simulink model "Sepic"  (R2019b)
settings: Solver=VariableStepAuto  StartTime=0.0  StopTime=0.02  RelTol=1e-7  AbsTol=1e-7
values from neighbouring files (symbols this model uses):
  HPFenable = 1    [SimMain.m]
  Ilim_sepic = 3.5    [SimMain.m]
  Ki_sepic = 1.1    [SimMain.m]
  Ku_sepic = 1    [SimMain.m]
  R1_sepic = 1    [SimMain.m]
  RL_sepic = 200    [SimMain.m]
  tau_PI_sepic = 0.5e-3    (= 0.0005)    [SimMain.m]
  U2_sepic = 20    [SimMain.m]
  w_Amplitude = 0.3    [SimMain.m]
libraries: fl_lib x14, nesl_utility x12, ee_lib x11, simulink x2, powerlib_meascontrol x2
settings Model: Creator=Job  LastModifiedBy=Job
settings SolverCC: AlgebraicLoopSolver=LineSearch  PositivePriorityOrder=on

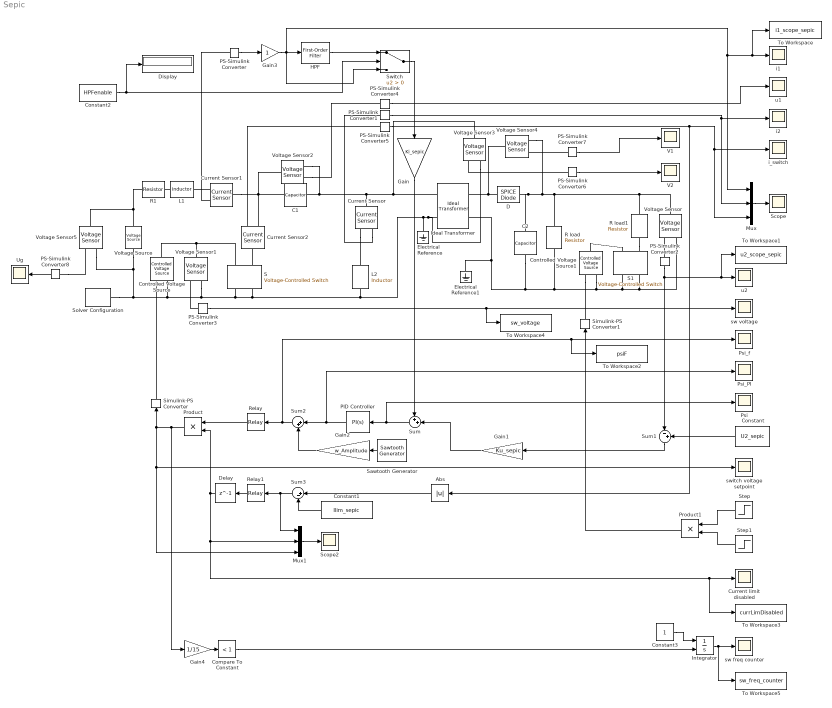
== system Sepic ==
  Abs : Abs
  C1 : ee_lib/Passive/Capacitor  cap_option=0  c=C1_sepic F  Cvec=[1e-05, 1e-06] F  Vvec=[0, 10] V  CV_table_symmetry=1  f_vec=[1, 10] kHz  DFext_vec=[.8, 1.2]  C_tol=0  enable_C_tol=0  tol_distribution=1  nSigma=4  r=1e-6 Ohm  g=0 1/Ohm  averaging_period=0 s  enable_operating_limits=0  operating_limit_action=2  max_working_voltage_range=[-25, 25] V  power_rating=1 W  enable_faults=0  fault_action=1  Cscale_faulted=100  R_faulted=1e-3 Ohm  G_faulted=0 1/Ohm  tau_fault=1e-3 s  enable_temporal_fault=0  t_fault=1 s  enable_behavioral_fault=0  max_permissible_voltage_range=[-100, 100] V  t_fail_on_voltage=1 s  i_specify=off  i_priority=None  i=0 A  i_nominal_specify=off  i_nominal_unit=A  i_nominal_value=1  v_specify=off  v_priority=None  v=0 V  v_nominal_specify=off  v_nominal_unit=V  v_nominal_value=1  vc_specify=off  vc_priority=High  vc=0 V  vc_nominal_specify=off  vc_nominal_unit=V  vc_nominal_value=1
      settings: SourceProductName=Simscape Electrical
  C2 : ee_lib/Passive/Capacitor  cap_option=0  c=C2_sepic F  Cvec=[1e-05, 1e-06] F  Vvec=[0, 10] V  CV_table_symmetry=1  f_vec=[1, 10] kHz  DFext_vec=[.8, 1.2]  C_tol=0  enable_C_tol=0  tol_distribution=1  nSigma=4  r=1e-6 Ohm  g=0 1/Ohm  averaging_period=0 s  enable_operating_limits=0  operating_limit_action=2  max_working_voltage_range=[-25, 25] V  power_rating=1 W  enable_faults=0  fault_action=1  Cscale_faulted=100  R_faulted=1e-3 Ohm  G_faulted=0 1/Ohm  tau_fault=1e-3 s  enable_temporal_fault=0  t_fault=1 s  enable_behavioral_fault=0  max_permissible_voltage_range=[-100, 100] V  t_fail_on_voltage=1 s  i_specify=off  i_priority=None  i=0 A  i_nominal_specify=off  i_nominal_unit=A  i_nominal_value=1  v_specify=off  v_priority=None  v=0 V  v_nominal_specify=off  v_nominal_unit=V  v_nominal_value=1  vc_specify=off  vc_priority=High  vc=0 V  vc_nominal_specify=off  vc_nominal_unit=V  vc_nominal_value=1
      settings: SourceProductName=Simscape Electrical
  Compare To Constant : simulink/Logic and Bit Operations/Compare To Constant  relop=<  const=1  OutDataTypeStr=boolean
  Constant : Constant  Value=U2_sepic
  Constant1 : Constant  Value=Ilim_sepic
  Constant2 : Constant  Value=HPFenable
  Constant3 : Constant
  Controlled Voltage Source : fl_lib/Electrical/Electrical Sources/Controlled Voltage Source
  Controlled Voltage Source1 : fl_lib/Electrical/Electrical Sources/Controlled Voltage Source
  Current Sensor : fl_lib/Electrical/Electrical Sensors/Current Sensor
  Current Sensor1 : fl_lib/Electrical/Electrical Sensors/Current Sensor
  Current Sensor2 : fl_lib/Electrical/Electrical Sensors/Current Sensor
  Current limit disabled : Scope
  D : ee_lib/Additional Components/SPICE Semiconductors/SPICE Diode  AREA=1.0 m^2  SCALE=1  IS=1e-14 A/m^2  RS=0.01 m^2*Ohm  N=1  C_param=1  CJO=0 F/m^2  VJ=1 V  M=0.5  FC=0.5  TT=0 s  RevBrk=1  BV=Inf V  IBV=1e-3 A/m^2  T_param=1  XTI=3.0  EG=1.11 eV  TFIXED=300.15 K  TMEAS=300.15 K  IC_given=1  V0=0 V  TOFFSET=0 K
      settings: SourceProductName=Simscape Electrical  SourceProductBaseCode=PS  InternalSimscapePortConfiguration="{\"Bottom\":[],\"Left\":[{\"id\":\"p\",\"label\":\"+\",\"type\":\"foundation.electrical.electrical\"}],\"Right\":[{\"id\":\"n\",\"label\":\"-\",\"type\":\"foundation.electrical.electrical\"}],\"Top\":[]}"
  Delay : Delay  DelayLength=1
  Display : Display
  Electrical Reference : fl_lib/Electrical/Electrical Elements/Electrical Reference
  Electrical Reference1 : fl_lib/Electrical/Electrical Elements/Electrical Reference
  Gain : Gain  Gain=Ki_sepic
  Gain1 : Gain  Gain=Ku_sepic
  Gain2 : Gain  Gain=w_Amplitude
  Gain3 : Gain
  Gain4 : Gain  Gain=1/15  OutDataTypeStr=uint8
  HPF : powerlib_meascontrol/Filters/First-Order Filter  FilterType=Highpass  Tc=tau_HPF_sepic  Ts=0  Initialize=off  Vac_Init=[0, 0, 60]  Vdc_Init=0  PlotResponse=off  FreqRange="[0,  200,  1]"
      settings: SourceProductName=Simscape Electrical
  Ideal Transformer : fl_lib/Electrical/Electrical Elements/Ideal Transformer  n=n_sepic  i1_specify=off  i1_priority=None  i1=0 A  i1_nominal_specify=off  i1_nominal_unit=A  i1_nominal_value=1  v1_specify=off  v1_priority=None  v1=0 V  v1_nominal_specify=off  v1_nominal_unit=V  v1_nominal_value=1  i2_specify=off  i2_priority=None  i2=0 A  i2_nominal_specify=off  i2_nominal_unit=A  i2_nominal_value=1  v2_specify=off  v2_priority=None  v2=0 V  v2_nominal_specify=off  v2_nominal_unit=V  v2_nominal_value=1
      settings: SourceProductName=Simscape  SourceProductBaseCode=SS
  Integrator : Integrator  ExternalReset=rising
  L1 : ee_lib/Passive/Inductor  l=L1_sepic H  L_tol=0  enable_L_tol=0  tol_distribution=1  nSigma=4  r=0.001 Ohm  g=1e-9 1/Ohm  enable_operating_limits=0  operating_limit_action=2  max_working_current=1 A  power_rating=1 W  enable_faults=0  fault_action=1  lambdaPercent=50  k_faulted=0.9999  turnsShort=0  openCct=0  groundShort=0  groundShortG=0 1/Ohm  tau_fault=1e-3 s  enable_temporal_fault=0  t_fault=1 s  enable_behavioral_fault=0  max_permissible_voltage=100 V  n_fail_on_voltage=1  max_permissible_current=1 A  t_fail_on_current=1 s  i_L_specify=off  i_L_priority=High  i_L=0 A  i_L_nominal_specify=off  i_L_nominal_unit=A  i_L_nominal_value=1
      settings: SourceProductName=Simscape Electrical
  L2 : ee_lib/Passive/Inductor  l=L2_sepic H  L_tol=0  enable_L_tol=0  tol_distribution=1  nSigma=4  r=0.001 Ohm  g=1e-9 1/Ohm  enable_operating_limits=0  operating_limit_action=2  max_working_current=1 A  power_rating=1 W  enable_faults=0  fault_action=1  lambdaPercent=50  k_faulted=0.9999  turnsShort=0  openCct=0  groundShort=0  groundShortG=0 1/Ohm  tau_fault=1e-3 s  enable_temporal_fault=0  t_fault=1 s  enable_behavioral_fault=0  max_permissible_voltage=100 V  n_fail_on_voltage=1  max_permissible_current=1 A  t_fail_on_current=1 s  i_L_specify=off  i_L_priority=High  i_L=0 A  i_L_nominal_specify=off  i_L_nominal_unit=A  i_L_nominal_value=1
      settings: SourceProductName=Simscape Electrical
  Mux : Mux  Inputs=3
  Mux1 : Mux  Inputs=3
  PID Controller : simulink/Continuous/PID Controller  Controller=PI  Form=Parallel  TimeDomain=Continuous-time  SampleTime=-1  IntegratorMethod=Forward Euler  FilterMethod=Forward Euler  ControllerParametersSource=internal  P=1  I=tau_PI_sepic  D=0  UseFilter=on  N=100  TunerSelectOption=Transfer Function Based (PID Tuner App)  InitialConditionSource=internal  InitialConditionForIntegrator=0  InitialConditionForFilter=0  DifferentiatorICPrevScaledInput=0  ExternalReset=none  TrackingMode=off  Kt=1  LimitOutput=off  UpperSaturationLimit=inf  LowerSaturationLimit=-inf  LinearizeAsGain=on  AntiWindupMode=none  Kb=1  POutMin=[]  POutMax=[]  IOutMin=[]  IOutMax=[]  DOutMin=[]  DOutMax=[]  NOutMin=[]  NOutMax=[]  SumOutMin=[]  SumOutMax=[]  SaturationOutMin=[]  SaturationOutMax=[]  PParamMin=[]  PParamMax=[]  IParamMin=[]  IParamMax=[]  DParamMin=[]  DParamMax=[]  NParamMin=[]  NParamMax=[]  KbParamMin=[]  KbParamMax=[]  KtParamMin=[]  KtParamMax=[]  KbOutMin=[]  KbOutMax=[]  KtOutMin=[]  KtOutMax=[]  IntegratorOutMin=[]  IntegratorOutMax=[]  FilterOutMin=[]  FilterOutMax=[]  SumI1OutMin=[]  SumI1OutMax=[]  SumI2OutMin=[]  SumI2OutMax=[]  SumI3OutMin=[]  SumI3OutMax=[]  SumI4OutMin=[]  SumI4OutMax=[]  SumDOutMin=[]  SumDOutMax=[]  DifferentiatorOutMin=[]  DifferentiatorOutMax=[]  FilterDiffOutCoefMin=[]  FilterDiffOutCoefMax=[]  ReciprocalOutMin=[]  ReciprocalOutMax=[]  SumDenOutMin=[]  SumDenOutMax=[]  SumNumOutMin=[]  SumNumOutMax=[]  DivideOutMin=[]  DivideOutMax=[]  IntegratorContinuousStateAttributes=''  IntegratorStateMustResolveToSignalObject=off  IntegratorRTWStateStorageClass=Auto  FilterContinuousStateAttributes=''  FilterStateMustResolveToSignalObject=off  FilterRTWStateStorageClass=Auto  ParallelPVariant=InternalParameters  IdealPVariant=Disabled  IVariant=InternalParameters  DVariant=Disabled  IntegratorVariant=Continuous  SatVariant=Disabled  AWVariant=Passthrough  PCopyVariant=Disabled  TRVariant=Disabled  FdbkBlocksVariant=Forward  IdealPFdbkVariant=Disabled  SatFdbkVariant=Disabled  DerivativeFilterVariant=Disabled  NVariant=Disabled  NCopyVariant=Disabled_SignalSpec  FilterICVariant=Disabled  IntegratorICVariant=InternalICs  ExternalResetVariant=Disabled  TRSumVariant=Passthrough  SumFdbkVariant=Disabled  SumVariant=Sum_PI
  PS-Simulink Converter{,1..8} (9 alike) : nesl_utility/PS-Simulink Converter  PhysicalDomain=network_engine_domain  SubClassName=ps_output  LeftPortType=input  RightPortType=output  PseudoPeriodic=off  Frequencies=[]  Unit=inherit  AffineConversion=off
  Product : Product
  Product1 : Product
  Psi : Scope
  Psi_PI : Scope
  Psi_f : Scope
  R load : ee_lib/Passive/Resistor  R=RL_sepic Ohm  R_tol=0.001  enable_R_tol=0  tol_distribution=1  nSigma=4  enable_operating_limits=0  operating_limit_action=2  max_working_voltage=100 V  power_rating=1 W  enable_faults=0  fault_action=1  R_faulted=inf Ohm  enable_temporal_fault=0  t_fault=1 s  enable_behavioral_fault=0  max_permissible_current=1 A  t_fail_on_current=1 s  noise_mode=0  sample_time=1e-3 s  repeatability=1  auto_seed=1005501763  user_seed=0  Tdevice=25 degC  alpha=3.93e-3 1/K  Tmeas=25 degC  thermal_mass=100 J/K  power_derating_T1=70 degC  power_derating_T2=155 degC  operating_temperature_range_vec=[-50, 150] degC  temperature_specify=off  temperature_priority=High  temperature=298.15 K  temperature_nominal_specify=off  temperature_nominal_unit=K  temperature_nominal_value=1
      settings: SourceProductName=Simscape Electrical
  R load1 : ee_lib/Passive/Resistor  R=22.222 Ohm  R_tol=0.001  enable_R_tol=0  tol_distribution=1  nSigma=4  enable_operating_limits=0  operating_limit_action=2  max_working_voltage=100 V  power_rating=1 W  enable_faults=0  fault_action=1  R_faulted=inf Ohm  enable_temporal_fault=0  t_fault=1 s  enable_behavioral_fault=0  max_permissible_current=1 A  t_fail_on_current=1 s  noise_mode=0  sample_time=1e-3 s  repeatability=1  auto_seed=2350272805  user_seed=0  Tdevice=25 degC  alpha=3.93e-3 1/K  Tmeas=25 degC  thermal_mass=100 J/K  power_derating_T1=70 degC  power_derating_T2=155 degC  operating_temperature_range_vec=[-50, 150] degC  temperature_specify=off  temperature_priority=High  temperature=298.15 K  temperature_nominal_specify=off  temperature_nominal_unit=K  temperature_nominal_value=1
      settings: SourceProductName=Simscape Electrical
  R1 : ee_lib/Passive/Resistor  R=R1_sepic Ohm  R_tol=0.1  enable_R_tol=0  tol_distribution=1  nSigma=4  enable_operating_limits=0  operating_limit_action=2  max_working_voltage=100 V  power_rating=1 W  enable_faults=0  fault_action=1  R_faulted=inf Ohm  enable_temporal_fault=0  t_fault=1 s  enable_behavioral_fault=0  max_permissible_current=1 A  t_fail_on_current=1 s  noise_mode=0  sample_time=1e-3 s  repeatability=1  auto_seed=551673987  user_seed=0  Tdevice=25 degC  alpha=3.93e-3 1/K  Tmeas=25 degC  thermal_mass=100 J/K  power_derating_T1=70 degC  power_derating_T2=155 degC  operating_temperature_range_vec=[-50, 150] degC  temperature_specify=off  temperature_priority=High  temperature=298.15 K  temperature_nominal_specify=off  temperature_nominal_unit=K  temperature_nominal_value=1
      settings: SourceProductName=Simscape Electrical
  Relay : Relay  OnSwitchValue=0.15  OffSwitchValue=-0.15  OnOutputValue=15
  Relay1 : Relay  OnSwitchValue=0  OffSwitchValue=-0.5  OnOutputValue=0  OffOutputValue=1
  S : ee_lib/Additional Components/SPICE Passives/Voltage-Controlled Switch  VT=1 V  VH=0 V  RON=0.0001 Ohm  ROFF=10e6 Ohm  IC_state=-1
      settings: SourceProductName=Simscape Electrical  SourceProductBaseCode=PS  InternalSimscapePortConfiguration="{\"Bottom\":[],\"Left\":[{\"id\":\"p1\",\"label\":\"1+\",\"type\":\"foundation.electrical.electrical\"},{\"id\":\"p2\",\"label\":\"2+\",\"type\":\"foundation.electrical.electrical\"}],\"Right\":[{\"id\":\"n1\",\"label\":\"1-\",\"type\":\"foundation.electrical.electrical\"},{\"id\":\"n2\",\"label\":\"2-\",\"type\":\"foundation.electrical.electrical\"}],\"Top\":[]}"
  S1 : ee_lib/Additional Components/SPICE Passives/Voltage-Controlled Switch  VT=1 V  VH=0 V  RON=0.0001 Ohm  ROFF=10e6 Ohm  IC_state=-1
      settings: SourceProductName=Simscape Electrical  SourceProductBaseCode=PS  InternalSimscapePortConfiguration="{\"Bottom\":[],\"Left\":[{\"id\":\"p1\",\"label\":\"1+\",\"type\":\"foundation.electrical.electrical\"},{\"id\":\"p2\",\"label\":\"2+\",\"type\":\"foundation.electrical.electrical\"}],\"Right\":[{\"id\":\"n1\",\"label\":\"1-\",\"type\":\"foundation.electrical.electrical\"},{\"id\":\"n2\",\"label\":\"2-\",\"type\":\"foundation.electrical.electrical\"}],\"Top\":[]}"
  Sawtooth Generator : powerlib_meascontrol/Pulse & Signal Generators/Sawtooth Generator  Freq=fg_sepic  Phase=0  Ts=0
      settings: SourceProductName=Simscape Electrical
  Scope : Scope
  Scope2 : Scope
  Simulink-PS Converter : nesl_utility/Simulink-PS Converter  PhysicalDomain=network_engine_domain  SubClassName=ps_input  LeftPortType=input  RightPortType=output  PseudoPeriodic=off  Frequencies=[]  NoiseDistribution=none  NoiseParameters=[]  Unit=1  AffineConversion=off  FilteringAndDerivatives=provide  SimscapeFilterOrder=1  InputFilterTimeConstant=0.001  UdotUserProvided=0
  Simulink-PS Converter1 : nesl_utility/Simulink-PS Converter  PhysicalDomain=network_engine_domain  SubClassName=ps_input  LeftPortType=input  RightPortType=output  PseudoPeriodic=off  Frequencies=[]  NoiseDistribution=none  NoiseParameters=[]  Unit=1  AffineConversion=off  FilteringAndDerivatives=provide  SimscapeFilterOrder=1  InputFilterTimeConstant=0.001  UdotUserProvided=0
  Solver Configuration : nesl_utility/Solver Configuration  PhysicalDomain=network_engine_domain  SubClassName=solver  LeftPortType=input  RightPortType=generic  Tones=[]  Harmonics=[]  SimulateNoise=off  Profile=off  UseLocalSampling=off  EnableSwitchedLinearOptims=on  FrequencyDomain=off  UseCCode=off  RelTol=0.001  AbsTol=1e-06  MinStep=1e-09  ToWorkspace=off  RevertToSquareIcSolve=off  NumHomotopyIterations=100  PhasorMode=off  PhasorModeNumHarmonics=1  DoDC=on  ResidualTolerance=1e-09  UseLocalSolver=off  LocalSolverChoice=NE_PARTITIONING_ADVANCER  LocalSolverSampleTime=1e-9  DoFixedCost=off  MaxNonlinIter=3  MaxModeIter=2  LinearAlgebra=auto  EquationFormulation=NE_TIME_EF  DelaysMemoryBudget=1024  AutomaticFiltering=off  FilteringTimeConstant=0.001  PartitionStorageMethod=AS_NEEDED  PartitionMemoryBudget=1024  PartitionMethod=ROBUST
  Step : Step  Time=0.01  After=5  SampleTime=0
  Step1 : Step  Time=0.015  Before=1  After=0  SampleTime=0
  Sum : Sum  Inputs=++|
  Sum1 : Sum  Inputs=|-+
  Sum2 : Sum  Inputs=|++
  Sum3 : Sum  Inputs=|+-
  Switch : Switch  Criteria=u2 > Threshold
  To Workspace : ToWorkspace  VariableName=i1_scope_sepic  SaveFormat=Timeseries  SampleTime=-1
  To Workspace1 : ToWorkspace  VariableName=u2_scope_sepic  SaveFormat=Timeseries  SampleTime=-1
  To Workspace2 : ToWorkspace  VariableName=psiF  SaveFormat=Timeseries  SampleTime=-1
  To Workspace3 : ToWorkspace  VariableName=currLimDisabled  SaveFormat=Timeseries  SampleTime=-1
  To Workspace4 : ToWorkspace  VariableName=sw_voltage  SaveFormat=Timeseries  SampleTime=-1
  To Workspace5 : ToWorkspace  VariableName=sw_freq_counter  SaveFormat=Timeseries  SampleTime=-1
  Ug : Scope
  V1 : Scope
  V2 : Scope
  Voltage Sensor{,1..5} (6 alike) : fl_lib/Electrical/Electrical Sensors/Voltage Sensor
  Voltage Source : ee_lib/Sources/Voltage Source  dc_voltage=Ug_sepic V  ac_voltage=4.5 V  ac_shift=0 rad  ac_frequency=100 Hz  noise_mode=0  PSD=0 V^2/Hz  repeatability=1  auto_seed=2816384857  user_seed=0  sample_time=1e-3 s  i_specify=off  i_priority=None  i=0 A  i_nominal_specify=off  i_nominal_unit=A  i_nominal_value=1  v_specify=off  v_priority=None  v=0 V  v_nominal_specify=off  v_nominal_unit=V  v_nominal_value=1
      settings: SourceProductName=Simscape Electrical
  i1 : Scope
  i2 : Scope
  i_switch : Scope
  sw freq counter : Scope
  sw voltage : Scope
  switch voltage setpoint : Scope
  u1 : Scope
  u2 : Scope
  wires:
  PS-Simulink Converter1/1 -> Mux/2, i2/1
  PS-Simulink Converter3/1 -> sw voltage/1, To Workspace4/1
  Gain3/1 -> Switch/3, HPF/1, Mux/1, To Workspace/1, i1/1
  PS-Simulink Converter/1 -> Gain3/1
  PS-Simulink Converter2/1 -> Sum1/1, To Workspace1/1, u2/1
  Gain1/1 -> Sum/2
  Gain/1 -> Sum/1
  Sum/1 -> Psi/1, PID Controller/1
  Sum1/1 -> Gain1/1
  Constant/1 -> Sum1/2
  PS-Simulink Converter4/1 -> u1/1
  PS-Simulink Converter5/1 -> Mux/3, i_switch/1, Abs/1
  Sawtooth Generator/1 -> Gain2/1
  Sum2/1 -> Relay/1, Psi_f/1, To Workspace2/1
  Gain2/1 -> Sum2/2
  PS-Simulink Converter7/1 -> V1/1
  PS-Simulink Converter6/1 -> V2/1
  Product/1 -> Simulink-PS Converter/1, Mux1/3, switch voltage setpoint/1, Gain4/1
  Constant1/1 -> Sum3/2
  Abs/1 -> Sum3/1
  Relay/1 -> Product/1
  Sum3/1 -> Mux1/1, Relay1/1
  Relay1/1 -> Delay/1
  Delay/1 -> Product/2, To Workspace3/1, Current limit disabled/1, Mux1/2
  Mux1/1 -> Scope2/1
  Mux/1 -> Scope/1
  Product1/1 -> Simulink-PS Converter1/1
  Step/1 -> Product1/1
  Step1/1 -> Product1/2
  PID Controller/1 -> Psi_PI/1, Sum2/1
  HPF/1 -> Switch/1
  Switch/1 -> Gain/1
  Constant2/1 -> Display/1, Switch/2
  PS-Simulink Converter8/1 -> Ug/1
  Gain4/1 -> Compare To Constant/1
  Constant3/1 -> Integrator/1
  Compare To Constant/1 -> Integrator/2
  Integrator/1 -> To Workspace5/1, sw freq counter/1
  connections:
  D/RConn1 -- Voltage Sensor4/RConn2 -- R load1/LConn1 -- Voltage Sensor/LConn1 -- R load/LConn1 -- C2/LConn1
  Voltage Sensor1/LConn1 -- Controlled Voltage Source/LConn1 -- S/LConn1
  S1/RConn1 -- S1/RConn2 -- Voltage Sensor/RConn2 -- Controlled Voltage Source1/RConn2 -- R load/RConn1 -- C2/RConn1 -- Ideal Transformer/RConn2 -- Electrical Reference1/LConn1
  C1/LConn1 -- Current Sensor1/LConn1 -- Voltage Sensor2/LConn1 -- Current Sensor2/RConn2
  Current Sensor/RConn1 -- PS-Simulink Converter1/LConn1
  Current Sensor1/RConn1 -- PS-Simulink Converter/LConn1
  PS-Simulink Converter3/LConn1 -- Voltage Sensor1/RConn1
  Voltage Source/LConn1 -- Voltage Sensor5/LConn1 -- R1/LConn1
  PS-Simulink Converter2/LConn1 -- Voltage Sensor/RConn1
  L1/LConn1 -- R1/RConn1
  Ideal Transformer/LConn1 -- Voltage Sensor3/LConn1 -- Current Sensor/LConn1 -- Voltage Sensor2/RConn2 -- C1/RConn1
  L2/RConn1 -- Electrical Reference/LConn1 -- Voltage Sensor3/RConn2 -- Ideal Transformer/LConn2 -- Voltage Sensor1/RConn2 -- Voltage Sensor5/RConn2 -- Voltage Source/RConn1 -- Solver Configuration/RConn1 -- Controlled Voltage Source/RConn2 -- S/RConn1 -- S/RConn2
  D/LConn1 -- Ideal Transformer/RConn1 -- Voltage Sensor4/LConn1
  Simulink-PS Converter/RConn1 -- Controlled Voltage Source/RConn1
  L1/RConn1 -- Current Sensor1/RConn2
  Current Sensor/RConn2 -- L2/LConn1
  Voltage Sensor2/RConn1 -- PS-Simulink Converter4/LConn1
  S/LConn2 -- Current Sensor2/LConn1
  Current Sensor2/RConn1 -- PS-Simulink Converter5/LConn1
  PS-Simulink Converter6/LConn1 -- Voltage Sensor3/RConn1
  PS-Simulink Converter7/LConn1 -- Voltage Sensor4/RConn1
  R load1/RConn1 -- S1/LConn2
  Controlled Voltage Source1/LConn1 -- S1/LConn1
  Controlled Voltage Source1/RConn1 -- Simulink-PS Converter1/RConn1
  PS-Simulink Converter8/LConn1 -- Voltage Sensor5/RConn1
